simulink model "ACC_upper_lower_controller"  (R2019a)
settings: Solver=VariableStepAuto  StartTime=0.0  StopTime=10.0  RelTol=1e-3
values from neighbouring files (symbols this model uses):
  c = 0.03    [ACC_initialization.m]
  ca = 0.5*1.225*9.95    (= 6.094375)    [ACC_initialization.m]
  coast_down_deceleration = 0.4    [ACC_initialization.m]
  d_desired = 50    [ACC_initialization.m]
  distance_sensor_range = 200    [ACC_initialization.m]
  h = 3*tau    (= 1.5)    [ACC_initialization.m]
  Kd_dist = 0.1    [ACC_initialization.m]
  Ki_vel = 0.3    [ACC_initialization.m]
  Kp_dist = 0.9    [ACC_initialization.m]
  Kp_vel = 1.0    (= 1)    [ACC_initialization.m]
  lambda = 0.9    [ACC_initialization.m]
  R = 3.25    [ACC_initialization.m]
  reff = 0.46    [ACC_initialization.m]
  v_desired = 20    [ACC_initialization.m]
  Weight = 1903    [ACC_initialization.m]
libraries: simulink x3
settings Model: Creator=Ajinkya Joglekar  LastModifiedBy=Ajinkya Joglekar

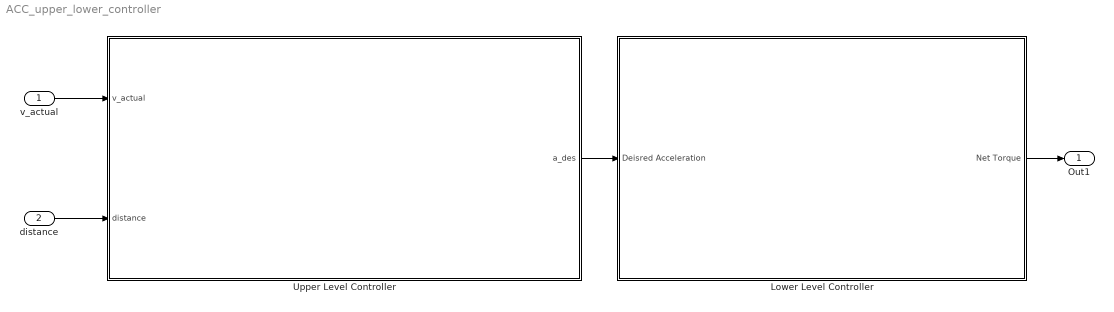
== system ACC_upper_lower_controller ==
  v_actual : Inport
  distance : Inport  Port=2
  Lower Level Controller : Subsystem
  Upper Level Controller : Subsystem
  Out1 : Outport
  wires:
  distance/1 -> Upper Level Controller/2(distance)
  v_actual/1 -> Upper Level Controller/1(v_actual)
  Lower Level Controller/1(Net Torque) -> Out1/1
  Upper Level Controller/1(a_des) -> Lower Level Controller/1(Deisred Acceleration)

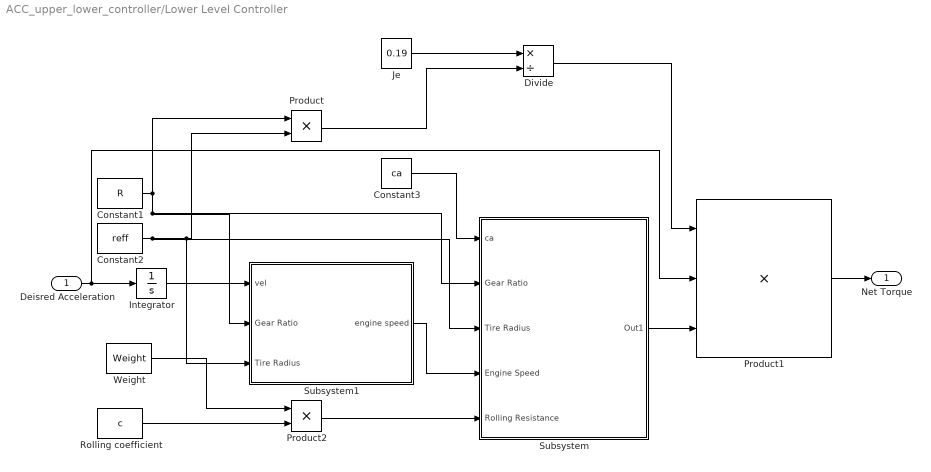
== system ACC_upper_lower_controller/Lower Level Controller ==
  Deisred Acceleration : Inport
  Constant1 : Constant  Value=R
  Constant2 : Constant  Value=reff
  Constant3 : Constant  Value=ca
  Divide : Product  Inputs=*/
  Integrator : Integrator
  Je : Constant  Value=0.19
  Product : Product
  Product1 : Product  Inputs=3
  Product2 : Product
  Rolling coefficient : Constant  Value=c
  Subsystem : Subsystem
  Subsystem1 : Subsystem
  Weight : Constant  Value=Weight
  Net Torque : Outport
  wires:
  Product/1 -> Divide/2
  Product1/1 -> Net Torque/1
  Divide/1 -> Product1/1
  Subsystem/1(Out1) -> Product1/3
  Constant2/1 -> Product/2, Subsystem1/3(Tire Radius), Subsystem/3(Tire Radius)
  Constant3/1 -> Subsystem/1(ca)
  Product2/1 -> Subsystem/5(Rolling Resistance)
  Je/1 -> Divide/1
  Integrator/1 -> Subsystem1/1(vel)
  Rolling coefficient/1 -> Product2/2
  Weight/1 -> Product2/1
  Subsystem1/1(engine speed) -> Subsystem/4(Engine Speed)
  Deisred Acceleration/1 -> Integrator/1, Product1/2
  Constant1/1 -> Subsystem/2(Gear Ratio), Subsystem1/2(Gear Ratio), Product/1

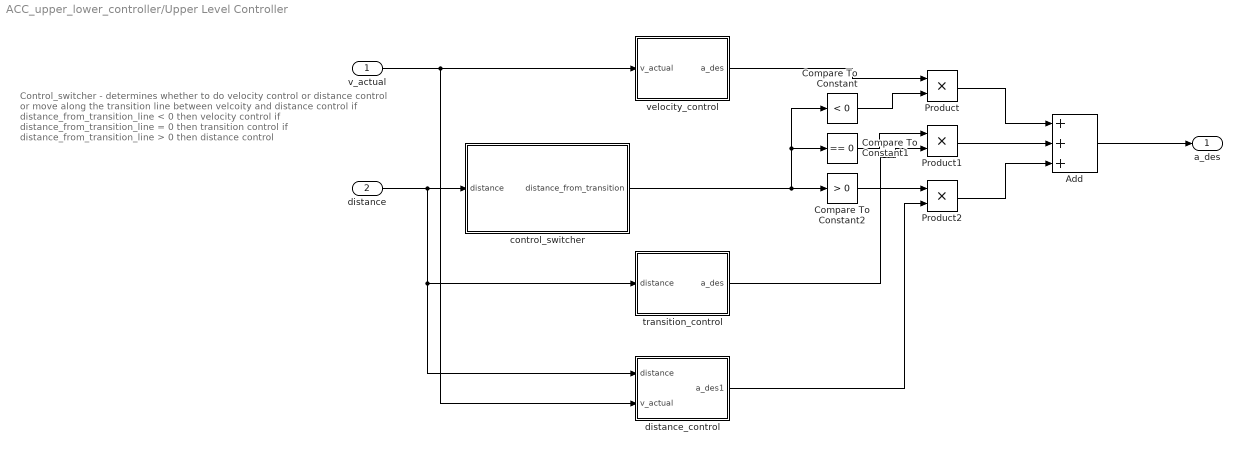
== system ACC_upper_lower_controller/Upper Level Controller ==
  note: Control_switcher - determines whether to do velocity control or distance control or move along the transition line between velcoity and distance control
      | if distance_from_transition_line < 0 then velocity control
      | if distance_from_transition_line = 0 then transition control
      | if distance_from_transition_line > 0 then distance control
  v_actual : Inport
  distance : Inport  Port=2
  Add : Sum  Inputs=3
  Compare To Constant : simulink/Logic and Bit Operations/Compare To Constant  relop=<  const=0  OutDataTypeStr=boolean
  Compare To Constant1 : simulink/Logic and Bit Operations/Compare To Constant  relop===  const=0  OutDataTypeStr=boolean
  Compare To Constant2 : simulink/Logic and Bit Operations/Compare To Constant  relop=>  const=0  OutDataTypeStr=boolean
  Product : Product
  Product1 : Product
  Product2 : Product
  control_switcher : Subsystem
  "distance_control " : Subsystem
  transition_control : Subsystem
  velocity_control : Subsystem
  a_des : Outport  VectorParamsAs1DForOutWhenUnconnected=on
  wires:
  Product2/1 -> Add/3
  control_switcher/1(distance_from_transition) -> Compare To Constant2/1, Compare To Constant1/1, Compare To Constant/1
  distance/1 -> transition_control/1(distance), "distance_control "/1(distance), control_switcher/1(distance)
  Product/1 -> Add/1
  velocity_control/1(a_des) -> Product/1
  "distance_control "/1(a_des1) -> Product2/2
  Add/1 -> a_des/1
  Compare To Constant2/1 -> Product2/1
  Compare To Constant/1 -> Product/2
  Product1/1 -> Add/2
  transition_control/1(a_des) -> Product1/2
  v_actual/1 -> "distance_control "/2(v_actual), velocity_control/1(v_actual)
  Compare To Constant1/1 -> Product1/1

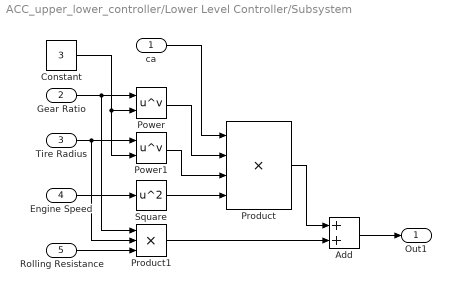
== system ACC_upper_lower_controller/Lower Level Controller/Subsystem ==
  ca : Inport
  Gear Ratio : Inport  Port=2
  Tire Radius : Inport  Port=3
  Engine Speed : Inport  Port=4
  Rolling Resistance : Inport  Port=5
  Add : Sum
  Constant : Constant  Value=3
  Power : Math  Operator=pow  SaturateOnIntegerOverflow=on
  Power1 : Math  Operator=pow  SaturateOnIntegerOverflow=on
  Product : Product  Inputs=4
  Product1 : Product  Inputs=3
  Square : Math  Operator=square  SaturateOnIntegerOverflow=on
  Out1 : Outport
  wires:
  Add/1 -> Out1/1
  Engine Speed/1 -> Square/1
  Product1/1 -> Add/2
  Product/1 -> Add/1
  Rolling Resistance/1 -> Product1/3
  Gear Ratio/1 -> Power/1, Product1/1
  Square/1 -> Product/4
  ca/1 -> Product/1
  Power1/1 -> Product/3
  Power/1 -> Product/2
  Tire Radius/1 -> Product1/2, Power1/1
  Constant/1 -> Power/2, Power1/2

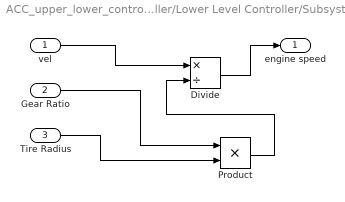
== system ACC_upper_lower_controller/Lower Level Controller/Subsystem1 ==
  vel : Inport
  Gear Ratio : Inport  Port=2
  Tire Radius : Inport  Port=3
  Divide : Product  Inputs=*/
  Product : Product
  engine speed : Outport
  wires:
  Gear Ratio/1 -> Product/1
  Tire Radius/1 -> Product/2
  vel/1 -> Divide/1
  Product/1 -> Divide/2
  Divide/1 -> engine speed/1

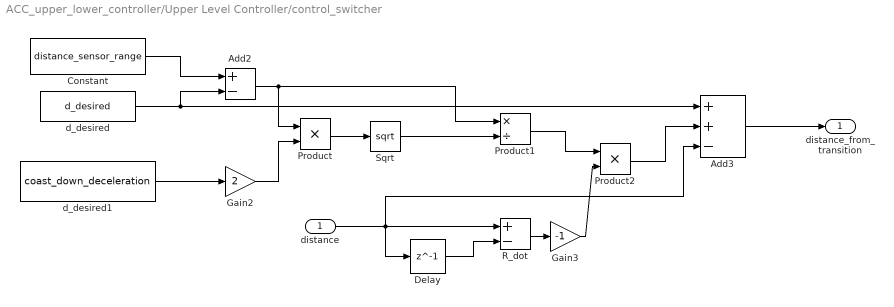
== system ACC_upper_lower_controller/Upper Level Controller/control_switcher ==
  distance : Inport
  Add2 : Sum  Inputs=+-
  Add3 : Sum  Inputs=++-
  Constant : Constant  Value=distance_sensor_range
  Delay : Delay  DelayLength=1
  Gain2 : Gain  Gain=2
  Gain3 : Gain  Gain=-1
  Product : Product
  Product1 : Product  Inputs=*/
  Product2 : Product
  R_dot : Sum  Inputs=+-
  Sqrt : Sqrt  SaturateOnIntegerOverflow=on
  d_desired : Constant  Value=d_desired
  d_desired1 : Constant  Value=coast_down_deceleration
  distance_from_transition : Outport  VectorParamsAs1DForOutWhenUnconnected=on
  wires:
  Constant/1 -> Add2/1
  d_desired/1 -> Add3/1, Add2/2
  d_desired1/1 -> Gain2/1
  Add2/1 -> Product/1, Product1/1
  Gain2/1 -> Product/2
  Product/1 -> Sqrt/1
  Sqrt/1 -> Product1/2
  distance/1 -> Delay/1, Add3/3, R_dot/1
  Delay/1 -> R_dot/2
  Product1/1 -> Product2/1
  R_dot/1 -> Gain3/1
  Gain3/1 -> Product2/2
  Product2/1 -> Add3/2
  Add3/1 -> distance_from_transition/1

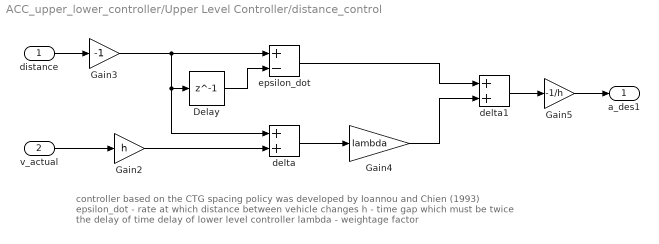
== system ACC_upper_lower_controller/Upper Level Controller/distance_control  ==
  note: controller based on the CTG spacing policy was developed by Ioannou and Chien (1993)
      | epsilon_dot - rate at which distance between vehicle changes
      | h - time gap which must be twice the delay of time delay of lower level controller
      | lambda - weightage factor
  distance : Inport
  v_actual : Inport  Port=2
  Delay : Delay  DelayLength=1
  Gain2 : Gain  Gain=h
  Gain3 : Gain  Gain=-1
  Gain4 : Gain  Gain=lambda
  Gain5 : Gain  Gain=-1/h
  delta : Sum
  delta1 : Sum
  epsilon_dot : Sum  Inputs=+-
  a_des1 : Outport  VectorParamsAs1DForOutWhenUnconnected=on
  wires:
  distance/1 -> Gain3/1
  Delay/1 -> epsilon_dot/2
  v_actual/1 -> Gain2/1
  Gain3/1 -> epsilon_dot/1, delta/1, Delay/1
  Gain2/1 -> delta/2
  delta/1 -> Gain4/1
  epsilon_dot/1 -> delta1/1
  Gain4/1 -> delta1/2
  delta1/1 -> Gain5/1
  Gain5/1 -> a_des1/1

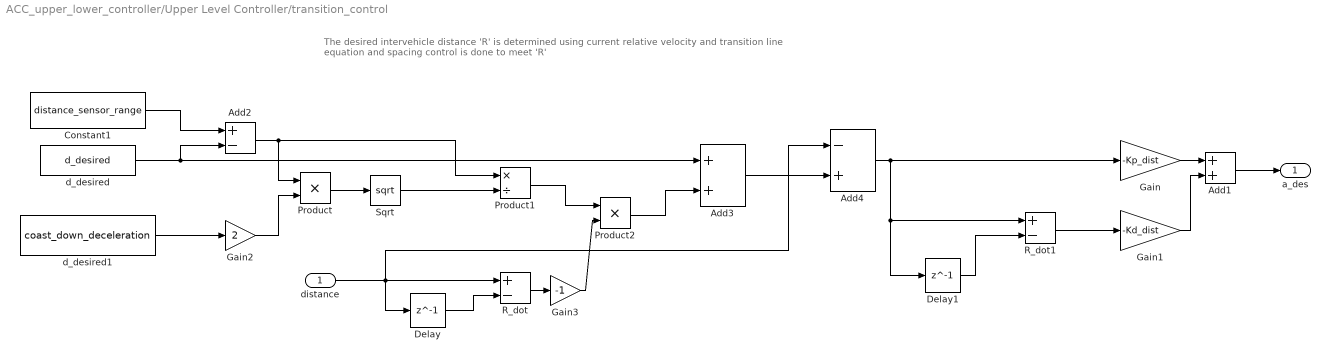
== system ACC_upper_lower_controller/Upper Level Controller/transition_control ==
  note: The desired intervehicle distance 'R' is determined using current relative velocity and transition line equation and spacing control is done to meet 'R'
  distance : Inport
  Add1 : Sum
  Add2 : Sum  Inputs=+-
  Add3 : Sum
  Add4 : Sum  Inputs=-+
  Constant1 : Constant  Value=distance_sensor_range
  Delay : Delay  DelayLength=1
  Delay1 : Delay  DelayLength=1
  Gain : Gain  Gain=-Kp_dist
  Gain1 : Gain  Gain=-Kd_dist
  Gain2 : Gain  Gain=2
  Gain3 : Gain  Gain=-1
  Product : Product
  Product1 : Product  Inputs=*/
  Product2 : Product
  R_dot : Sum  Inputs=+-
  R_dot1 : Sum  Inputs=+-
  Sqrt : Sqrt  SaturateOnIntegerOverflow=on
  d_desired : Constant  Value=d_desired
  d_desired1 : Constant  Value=coast_down_deceleration
  a_des : Outport  VectorParamsAs1DForOutWhenUnconnected=on
  wires:
  Gain/1 -> Add1/1
  Add1/1 -> a_des/1
  Gain1/1 -> Add1/2
  Add4/1 -> Delay1/1, R_dot1/1, Gain/1
  d_desired/1 -> Add3/1, Add2/2
  Add2/1 -> Product/1, Product1/1
  R_dot/1 -> Gain3/1
  Product/1 -> Sqrt/1
  Gain3/1 -> Product2/2
  Sqrt/1 -> Product1/2
  Delay/1 -> R_dot/2
  distance/1 -> Delay/1, Add4/1, R_dot/1
  d_desired1/1 -> Gain2/1
  Product1/1 -> Product2/1
  Gain2/1 -> Product/2
  Constant1/1 -> Add2/1
  Product2/1 -> Add3/2
  Add3/1 -> Add4/2
  R_dot1/1 -> Gain1/1
  Delay1/1 -> R_dot1/2

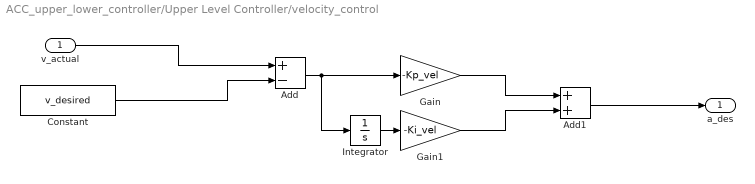
== system ACC_upper_lower_controller/Upper Level Controller/velocity_control ==
  v_actual : Inport
  Add : Sum  Inputs=+-
  Add1 : Sum
  Constant : Constant  Value=v_desired
  Gain : Gain  Gain=-Kp_vel
  Gain1 : Gain  Gain=-Ki_vel
  Integrator : Integrator
  a_des : Outport  VectorParamsAs1DForOutWhenUnconnected=on
  wires:
  v_actual/1 -> Add/1
  Add/1 -> Gain/1, Integrator/1
  Gain1/1 -> Add1/2
  Constant/1 -> Add/2
  Add1/1 -> a_des/1
  Gain/1 -> Add1/1
  Integrator/1 -> Gain1/1
